simulink model "dsogi_pll_3ph_top"  (R2024b)
settings: configuration reference "SharedConfig" (kept outside this file)
undefined symbols (not defined in the file or in its folder): ang2, freq2
libraries: simulink x1
settings Model: DataDictionary=dictionary.sldd  Creator=ASUSTUF  LastModifiedBy=Angel
settings ConfigSetRef: SourceName=SharedConfig

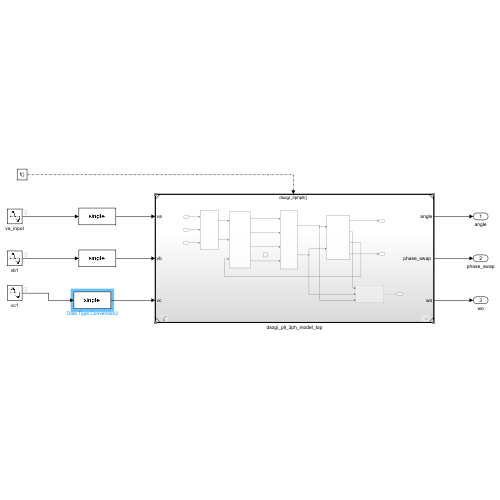
[thumbnail: Simulink's stored preview of the top-level diagram]
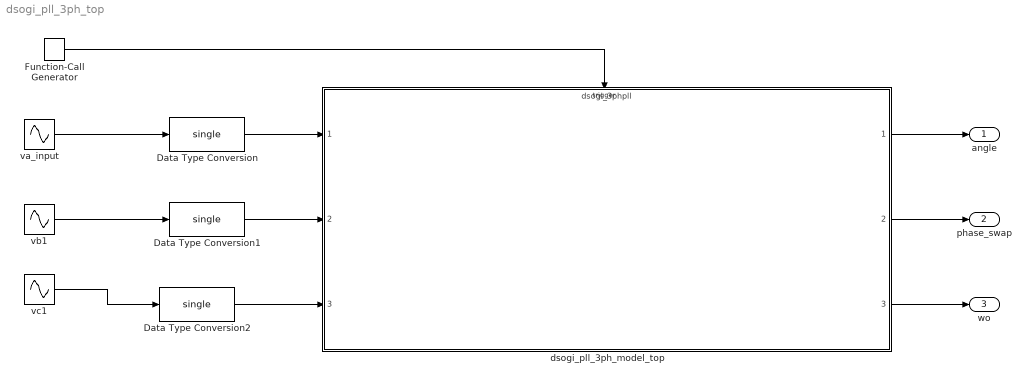
== system dsogi_pll_3ph_top ==
  Data Type Conversion : DataTypeConversion  OutDataTypeStr=single  SaturateOnIntegerOverflow=off  RndMeth=Floor
  Data Type Conversion1 : DataTypeConversion  OutDataTypeStr=single  SaturateOnIntegerOverflow=off  RndMeth=Floor
  Data Type Conversion2 : DataTypeConversion  OutDataTypeStr=single  SaturateOnIntegerOverflow=off  RndMeth=Floor
  Function-Call Generator : simulink/Ports & Subsystems/Function-Call Generator  sample_time=1/10e3  numberOfIterations=1  DisallowWideOutput=off
  dsogi_pll_3ph_model_top : ModelReference  ModelNameDialog=dsogi_3phpll.slx  SimulationMode=Normal  ModelReferenceVersion=1.15  TriggerPortName=function  TriggerPortTriggerType=function-call  TriggerPortStatesWhenEnabling=held
  va_input : Sin  Frequency=2*pi*freq2  Phase=ang2  SampleTime=1/10e3
  vb1 : Sin  Frequency=2*pi*freq2  Phase=-pi*12/18+ang2  SampleTime=1/10e3
  vc1 : Sin  Frequency=2*pi*freq2  Phase=pi*12/18+ang2  SampleTime=1/10e3
  angle : Outport
  phase_swap : Outport  Port=2
  wo : Outport  Port=3
  wires:
  dsogi_pll_3ph_model_top/2 -> phase_swap/1
  dsogi_pll_3ph_model_top/1 -> angle/1
  dsogi_pll_3ph_model_top/3 -> wo/1
  Function-Call Generator/1 -> dsogi_pll_3ph_model_top/Trigger
  vb1/1 -> Data Type Conversion1/1
  vc1/1 -> Data Type Conversion2/1
  va_input/1 -> Data Type Conversion/1
  Data Type Conversion/1 -> dsogi_pll_3ph_model_top/1
  Data Type Conversion1/1 -> dsogi_pll_3ph_model_top/2
  Data Type Conversion2/1 -> dsogi_pll_3ph_model_top/3
